simulink model "Question10"  (R2020a)
settings: Solver=VariableStepAuto  StartTime=0.0  StopTime=10.0  RelTol=1e-3
undefined symbols (not defined in the file or in its folder): V
libraries: simulink x3
settings Model: Creator=aishw  LastModifiedBy=aishw

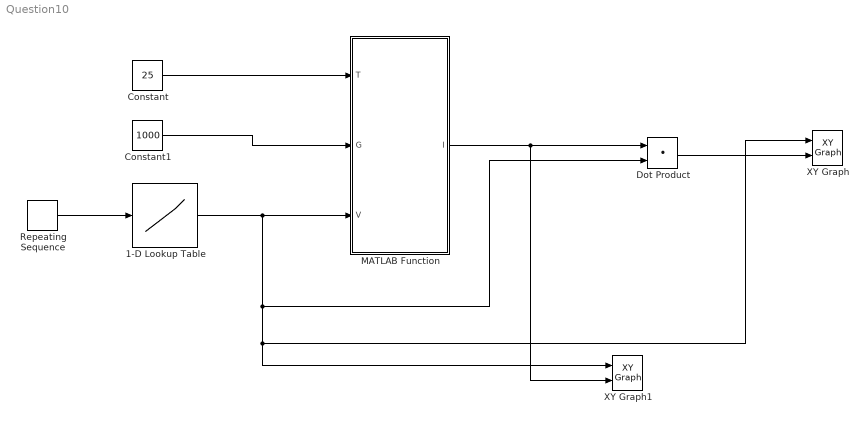
== system Question10 ==
  1-D Lookup Table : Lookup_n-D  NumberOfTableDimensions=1  BreakpointsForDimension1=[1:330]  Table=V([1:330])  InternalRulePriority=Speed  RndMeth=Simplest  InputSameDT=on
  Constant : Constant  Value=25
  Constant1 : Constant  Value=1000
  Dot Product : DotProduct  InputSameDT=on  OutDataTypeStr=Inherit: Inherit via internal rule
  MATLAB Function : MATLAB Function  TreatAsAtomicUnit=on
  Repeating Sequence : simulink/Sources/Repeating Sequence  rep_seq_t=[0 2]  rep_seq_y=[0 330]
  XY Graph : simulink/Sinks/XY Graph  xmin=0  xmax=50  ymin=0  ymax=200  st=1
  XY Graph1 : simulink/Sinks/XY Graph  xmin=0  xmax=50  ymin=0  ymax=10  st=1
  wires:
  Repeating Sequence/1 -> 1-D Lookup Table/1
  Constant1/1 -> MATLAB Function/2(G)
  Constant/1 -> MATLAB Function/1(T)
  MATLAB Function/1(I) -> Dot Product/1, XY Graph1/2
  1-D Lookup Table/1 -> Dot Product/2, XY Graph/1, XY Graph1/1, MATLAB Function/3(V)
  Dot Product/1 -> XY Graph/2

== matlab function Question10/MATLAB Function ==
  data: T input; I output; G input; V input
function I = fcn(T,G,V)

K = 1.38065e-23;
q = 1.602e-19;
Iscn = 8.21;
Vocn = 32.9;
Kv = -0.123;
Ki = 0.0032;
Ns = 54;
T = T+273;
Tn = 25+273;
Gn = 1050;
a = 1.3;
Eg = 1.12;
Rs = 0.221;
Rp = 415.405;
I = 0;

Vtn = Ns*(K*Tn/q);

Ion = Iscn/((exp(Vocn/(a*Vtn)))-1);

Io_part = ((q*Eg/(a*K))*((1/Tn)-(1/T)));
Io = Ion*((Tn/T)^3)*exp(Io_part);
Ipvn = Iscn;
Ipv = (Ipvn + Ki*(T-Tn))*(G/Gn);
Vt = Ns*(K*T/q);
I_part = Io*(exp((V+(I*Rs))/(Vt*a))-1) + ((V+(Rs*I))/Rp);
I = Ipv -I_part;
